simulink model "test_motor_control"  (R2016a)
settings: Solver=VariableStepAuto  StartTime=0.0  StopTime=0.25  RelTol=1e-3
settings Model: Creator=Matias  LastModifiedBy=Matias
settings DataIOCC: SaveFormat=Structure

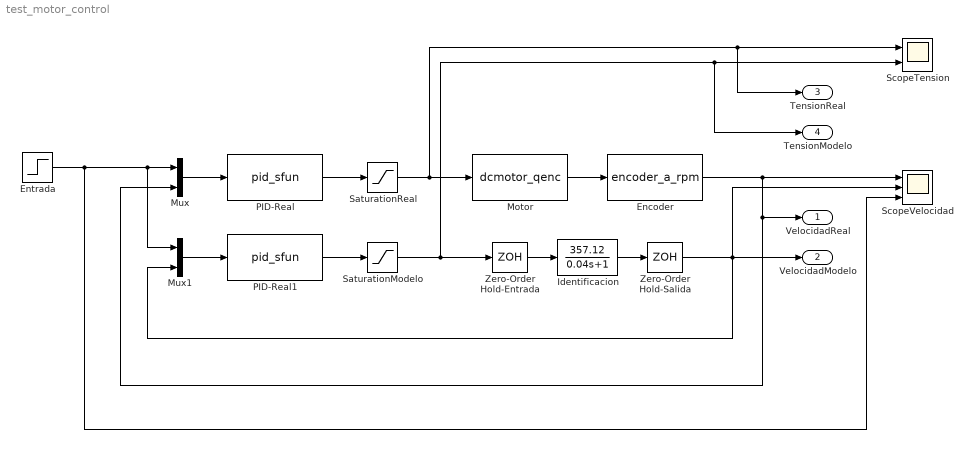
== system test_motor_control ==
  Encoder : S-Function  FunctionName=encoder_a_rpm  Parameters=0.00001, 0.005,150  SFunctionDeploymentMode=off  EnableBusSupport=off
  Entrada : Step  Time=0  After=4000  SampleTime=0
  Identificacion : TransferFcn  Numerator=[357.12]  Denominator=[0.04 1]
  Motor : S-Function  FunctionName=dcmotor_qenc  Parameters=150  SFunctionDeploymentMode=off  EnableBusSupport=off
  Mux : Mux  Inputs=2
  Mux1 : Mux  Inputs=2
  PID-Real : S-Function  FunctionName=pid_sfun  Parameters=0.005 25 0.00125 0.005 1/10  SFunctionDeploymentMode=off  EnableBusSupport=off
  PID-Real1 : S-Function  FunctionName=pid_sfun  Parameters=0.008 25 0.00125 0.005 1/10  SFunctionDeploymentMode=off  EnableBusSupport=off
  "SaturationModelo " : Saturate  UpperLimit=30  LowerLimit=-30
  SaturationReal : Saturate  UpperLimit=30  LowerLimit=-30
  ScopeTension : Scope  NumInputPorts=2
  ScopeVelocidad : Scope  NumInputPorts=3
  Zero-Order Hold-Entrada : ZeroOrderHold  SampleTime=0.005
  Zero-Order Hold-Salida : ZeroOrderHold  SampleTime=0.005
  VelocidadReal : Outport
  "VelocidadModelo " : Outport  Port=2
  TensionReal : Outport  Port=3
  TensionModelo : Outport  Port=4
  wires:
  Motor/1 -> Encoder/1
  Identificacion/1 -> Zero-Order Hold-Salida/1
  Encoder/1 -> Mux/2, VelocidadReal/1, ScopeVelocidad/1
  Zero-Order Hold-Salida/1 -> Mux1/2, "VelocidadModelo "/1, ScopeVelocidad/2
  SaturationReal/1 -> TensionReal/1, ScopeTension/1, Motor/1
  "SaturationModelo "/1 -> TensionModelo/1, ScopeTension/2, Zero-Order Hold-Entrada/1
  Entrada/1 -> ScopeVelocidad/3, Mux1/1, Mux/1
  PID-Real1/1 -> "SaturationModelo "/1
  Mux1/1 -> PID-Real1/1
  Zero-Order Hold-Entrada/1 -> Identificacion/1
  PID-Real/1 -> SaturationReal/1
  Mux/1 -> PID-Real/1
